simulink model "BPSK"  (R2018b)
settings: Solver=FixedStepAuto  StartTime=0.0  StopTime=10.0  FixedStep=0.01  RelTol=1e-3
settings Model: Creator=root  LastModifiedBy=root

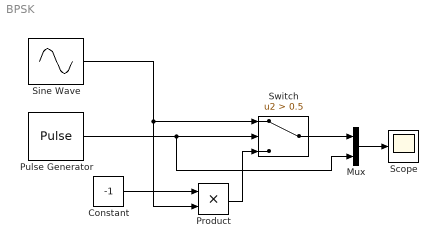
== system BPSK ==
  Constant : Constant  Value=-1
  Mux : Mux  Inputs=2
  Product : Product
  Pulse Generator : DiscretePulseGenerator  PulseType=Time based  PulseWidth=50
  Scope : Scope
  Sine Wave : Sin  Frequency=2*pi*2  SampleTime=0.01
  Switch : Switch  Criteria=u2 > Threshold  Threshold=0.5
  wires:
  Constant/1 -> Product/1
  Sine Wave/1 -> Switch/1, Product/2
  Product/1 -> Switch/3
  Pulse Generator/1 -> Mux/2, Switch/2
  Switch/1 -> Mux/1
  Mux/1 -> Scope/1
